simulink model "szybkozmienny_interpolacja"  (R2017b)
settings: Solver=FixedStepDiscrete  StartTime=0.0  StopTime=0.0  RelTol=1e-3
libraries: CPOiS_SourcesSinks x4, CPOiS_DataManipulation x1
settings Model: Creator=alis  LastModifiedBy=alis

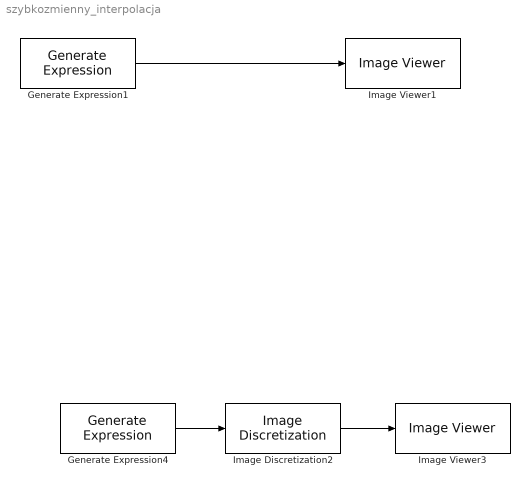
== system szybkozmienny_interpolacja ==
  Generate Expression1 : CPOiS_SourcesSinks/Generate Expression  Width=256  Height=256  Expression=255.*(mod(W,4)>1)
      settings: SourceProductName=CPOiS - Digital image and signal processing
  Generate Expression4 : CPOiS_SourcesSinks/Generate Expression  Width=256  Height=256  Expression=255.*(mod(W,4)>1)
      settings: SourceProductName=CPOiS - Digital image and signal processing
  Image Discretization2 : CPOiS_DataManipulation/Image Discretization  factor=8
      settings: SourceProductName=CPOiS - Digital image and signal processing
  Image Viewer1 : CPOiS_SourcesSinks/Image Viewer
      settings: SourceProductName=CPOiS - Digital image and signal processing
  Image Viewer3 : CPOiS_SourcesSinks/Image Viewer
      settings: SourceProductName=CPOiS - Digital image and signal processing
  wires:
  Generate Expression1/1 -> Image Viewer1/1
  Image Discretization2/1 -> Image Viewer3/1
  Generate Expression4/1 -> Image Discretization2/1
